simulink model "lab5"  (Simulink 8.1)
settings: Solver=ode3  StartTime=0.0  StopTime=t  FixedStep=dt  RelTol=1e-3
values from neighbouring files (symbols this model uses):
  A = 0.05    [lab5.m]
  b = 2000    [lab5.m]
  g = 9.81    [lab5.m]
  k1 = 20000    [lab5.m]
  k2 = 200000    [lab5.m]
  m1 = 400    [lab5.m]
  m2 = 50    [lab5.m]
  Td = 5    [lab5.m]
settings Model: Creator=Jan  LastModifiedBy=Jan
settings DataIOCC: SignalLoggingSaveFormat=Dataset
settings OptimizationCC: ExpressionDepthLimit=128
settings DebuggingCC: FcnCallInpInsideContextMsg=EnableAllAsError
settings GRTTargetCC: CombineOutputUpdateFcns=on  GRTInterface=off

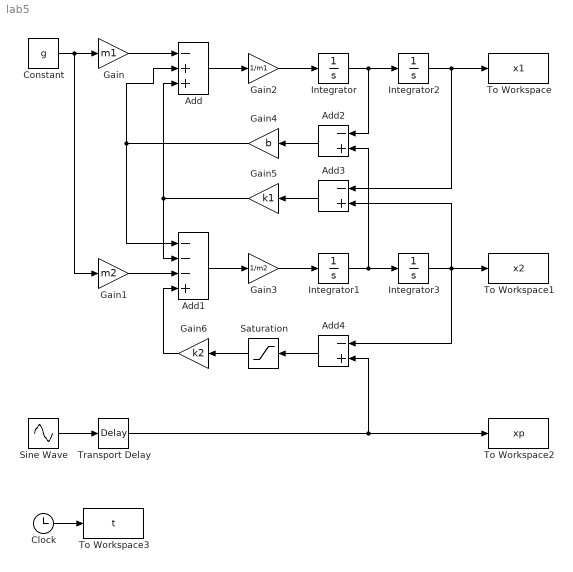
== system lab5 ==
  Add : Sum  Inputs=-++
  Add1 : Sum  Inputs=---+
  Add2 : Sum  Inputs=-+
  Add3 : Sum  Inputs=-+
  Add4 : Sum  Inputs=-+
  Clock : Clock
  Constant : Constant  Value=g
  Gain : Gain  Gain=m1
  Gain1 : Gain  Gain=m2
  Gain2 : Gain  Gain=1/m1
  Gain3 : Gain  Gain=1/m2
  Gain4 : Gain  Gain=b
  Gain5 : Gain  Gain=k1
  Gain6 : Gain  Gain=k2
  Integrator{,1..3} (4 alike) : Integrator
  Saturation : Saturate  UpperLimit=Inf  LowerLimit=0
  Sine Wave : Sin  Amplitude=A  SampleTime=0
  To Workspace : ToWorkspace  VariableName=x1  SampleTime=-1
  To Workspace1 : ToWorkspace  VariableName=x2  SampleTime=-1
  To Workspace2 : ToWorkspace  VariableName=xp  SampleTime=-1
  To Workspace3 : ToWorkspace  VariableName=t  SampleTime=-1
  Transport Delay : TransportDelay  DelayTime=Td
  wires:
  Constant/1 -> Gain1/1, Gain/1
  Gain/1 -> Add/1
  Gain1/1 -> Add1/3
  Gain4/1 -> Add1/1, Add/2
  Gain5/1 -> Add/3, Add1/2
  Add/1 -> Gain2/1
  Add1/1 -> Gain3/1
  Add3/1 -> Gain5/1
  Add2/1 -> Gain4/1
  Gain2/1 -> Integrator/1
  Gain3/1 -> Integrator1/1
  Integrator/1 -> Add2/1, Integrator2/1
  Integrator1/1 -> Add2/2, Integrator3/1
  Integrator2/1 -> Add3/1, To Workspace/1
  Integrator3/1 -> Add4/1, Add3/2, To Workspace1/1
  Gain6/1 -> Add1/4
  Saturation/1 -> Gain6/1
  Add4/1 -> Saturation/1
  Sine Wave/1 -> Transport Delay/1
  Transport Delay/1 -> Add4/2, To Workspace2/1
  Clock/1 -> To Workspace3/1
